simulink library "slrtencoderlib"  (R2022a)
settings: Solver=VariableStepAuto  StartTime=0.0  StopTime=10.0  RelTol=1e-3
libraries: simulink x3
settings Model: Creator=chrisz  LastModifiedBy=chrisz
settings SolverCC: MaxZcPerStep=1

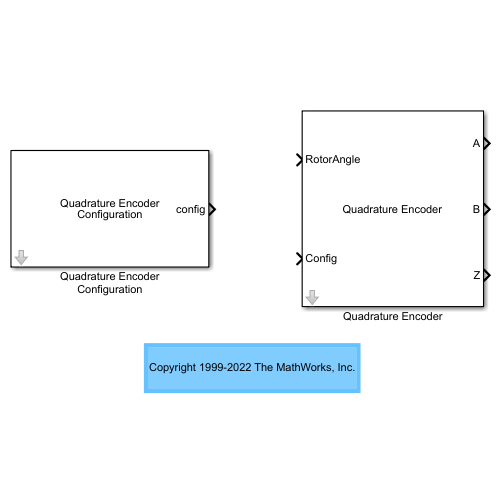
[thumbnail: Simulink's stored preview of the top-level diagram]
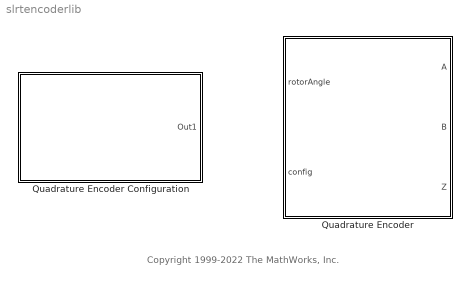
== system slrtencoderlib ==
  note: Copyright 1999-2022 The MathWorks, Inc.
  Quadrature Encoder : Subsystem  mask(Quadrature Encoder){}
      mask help: HDL coder compatible implementation of quadrature encoder. This model simulates FPGA clock level operations and is not suited for desktop simulation other than for validating the real-time model is accurate. It should primarily be used when generating HDL for real-time systems. Use standard blocks for desktop simulation.
      mask Display:
      | disp('Quadrature Encoder');
      | port_label('input',1,'RotorAngle');
      | port_label('input',2,'Config');
      | port_label('output',1,'A');
      | port_label('output',2,'B');
      | port_label('output',3,'Z');
  Quadrature Encoder Configuration : Subsystem  mask(Quadrature Encoder Configuration){NPulses=2000, zOffset=0, Ts=1e-6}
      mask prompts: NPulses "Pulses per revolution:"; zOffset "Index pulse offset relative to shaft initial angle (deg):"; Ts "Sample time (s):"
      mask help: Configuration block for HDL coder compatible implementation of quadrature encoder. This block intends to be used for configuring the corresponding encoder block on FPGA.
      mask Display:
      | disp('Quadrature Encoder\nConfiguration')
      | port_label('output', 1, 'config')

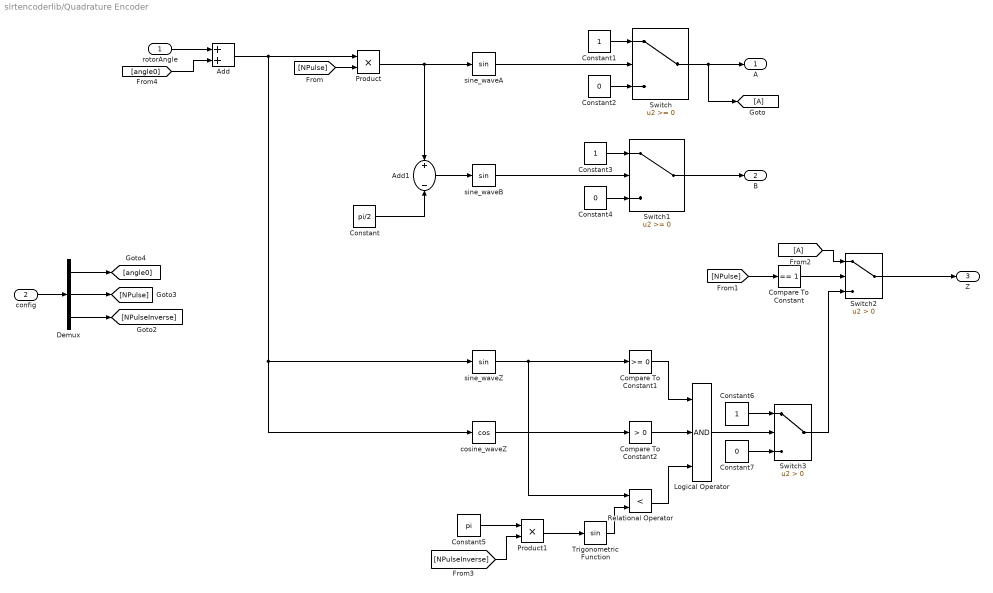
== system slrtencoderlib/Quadrature Encoder ==
  rotorAngle : Inport
  config : Inport  Port=2
  Add : Sum
  Add1 : Sum  Inputs=+-
  Compare To Constant : simulink/Logic and Bit Operations/Compare To Constant  relop===  const=1  OutDataTypeStr=boolean
  Compare To Constant1 : simulink/Logic and Bit Operations/Compare To Constant  relop=>=  const=0  OutDataTypeStr=boolean
  Compare To Constant2 : simulink/Logic and Bit Operations/Compare To Constant  relop=>  const=0  OutDataTypeStr=boolean
  Constant : Constant  Value=pi/2  OutDataTypeStr=single  SampleTime=-1
  Constant1 : Constant  OutDataTypeStr=boolean  SampleTime=-1
  Constant2 : Constant  Value=0  OutDataTypeStr=boolean  SampleTime=-1
  Constant3 : Constant  OutDataTypeStr=boolean  SampleTime=-1
  Constant4 : Constant  Value=0  OutDataTypeStr=boolean  SampleTime=-1
  Constant5 : Constant  Value=pi  OutDataTypeStr=single  SampleTime=-1
  Constant6 : Constant  OutDataTypeStr=uint64  SampleTime=-1
  Constant7 : Constant  Value=0  OutDataTypeStr=boolean  SampleTime=-1
  Demux : Demux  Outputs=3
  From2 : From
  Goto : Goto
  Logical Operator : Logic  Inputs=3  AllPortsSameDT=off  OutDataTypeStr=boolean
  Product : Product  OutDataTypeStr=single
  Product1 : Product
  Relational Operator : RelationalOperator  Operator=<  OutDataTypeStr=boolean  RndMeth=Simplest  InputSameDT=off
  Switch : Switch  SaturateOnIntegerOverflow=off  InputSameDT=off
  Switch1 : Switch  SaturateOnIntegerOverflow=off  InputSameDT=off
  Switch2 : Switch  Criteria=u2 > Threshold  OutDataTypeStr=boolean  SaturateOnIntegerOverflow=off  InputSameDT=off
  Switch3 : Switch  Criteria=u2 > Threshold  SaturateOnIntegerOverflow=off  InputSameDT=off
  Trigonometric Function : Trigonometry
  cosine_waveZ : Trigonometry  Operator=cos
  sine_waveA : Trigonometry
  sine_waveB : Trigonometry
  sine_waveZ : Trigonometry
  A : Outport
  B : Outport  Port=2
  Z : Outport  Port=3
  wires:
  Product/1 -> Add1/1, sine_waveA/1
  rotorAngle/1 -> Add/1
  [angle0] -> Add/2
  Add/1 -> cosine_waveZ/1, sine_waveZ/1, Product/1
  Constant/1 -> Add1/2
  Add1/1 -> sine_waveB/1
  sine_waveA/1 -> Switch/2
  Constant1/1 -> Switch/1
  Constant2/1 -> Switch/3
  Switch/1 -> Goto/1, A/1
  Constant4/1 -> Switch1/3
  Constant3/1 -> Switch1/1
  sine_waveB/1 -> Switch1/2
  Switch1/1 -> B/1
  Compare To Constant/1 -> Switch2/2
  [NPulse] -> Product/2
  [NPulse] -> Compare To Constant/1
  From2/1 -> Switch2/1
  Switch2/1 -> Z/1
  sine_waveZ/1 -> Relational Operator/1, Compare To Constant1/1
  cosine_waveZ/1 -> Compare To Constant2/1
  Constant5/1 -> Product1/1
  [NPulseInverse] -> Product1/2
  Product1/1 -> Trigonometric Function/1
  Trigonometric Function/1 -> Relational Operator/2
  Compare To Constant1/1 -> Logical Operator/1
  Compare To Constant2/1 -> Logical Operator/2
  Relational Operator/1 -> Logical Operator/3
  Logical Operator/1 -> Switch3/2
  Constant7/1 -> Switch3/3
  Constant6/1 -> Switch3/1
  Switch3/1 -> Switch2/3
  config/1 -> Demux/1
  Demux/2 -> [NPulse]
  Demux/1 -> [angle0]
  Demux/3 -> [NPulseInverse]

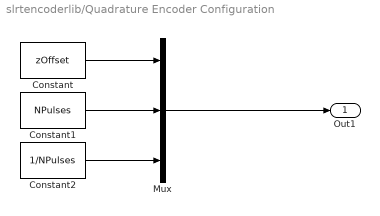
== system slrtencoderlib/Quadrature Encoder Configuration ==
  Constant : Constant  Value=zOffset  OutDataTypeStr=single  SampleTime=Ts
  Constant1 : Constant  Value=NPulses  OutDataTypeStr=single  SampleTime=Ts
  Constant2 : Constant  Value=1/NPulses  OutDataTypeStr=single  SampleTime=Ts
  Mux : Mux  Inputs=3
  Out1 : Outport
  wires:
  Mux/1 -> Out1/1
  Constant1/1 -> Mux/2
  Constant/1 -> Mux/1
  Constant2/1 -> Mux/3
